simulink library "MicDiagWithdBFSOutput"  (R2022b)
settings: Solver=VariableStepAuto  StartTime=0.0  StopTime=10.0  RelTol=1e-3
values from neighbouring files (symbols this model uses):
  numMicIn = 2    [PhaseDetector_init.m]
undefined symbols (not defined in the file or in its folder): framesize
libraries: RTC x2, FeaturePath x1
settings Model: Creator=pk47312  LastModifiedBy=jk1043656
settings SolverCC: AlgebraicLoopSolver=TrustRegion
settings DebuggingCC: UnconnectedInputMsg=warning  UnconnectedOutputMsg=warning  UnconnectedLineMsg=warning  SFMachineParentedDataDiag=warning
settings ModelReferenceCC: EnableRefExpFcnMdlSchedulingChecks=on
settings RTWCC: DLArmComputeVersion=19.05

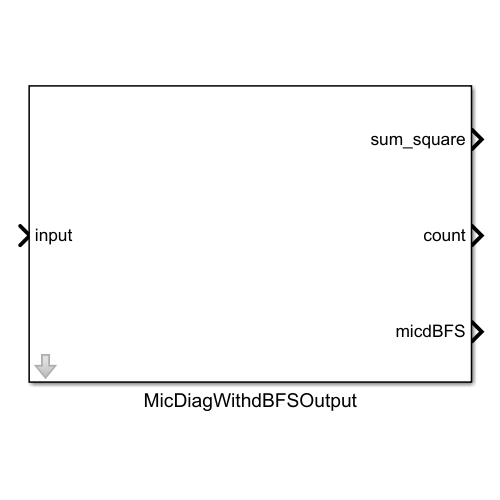
[thumbnail: Simulink's stored preview of the top-level diagram]
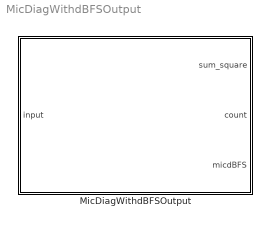
== system MicDiagWithdBFSOutput ==
  MicDiagWithdBFSOutput : Subsystem  mask{numMicIn=numMicIn, framesize=framesize}
      mask prompts: numMicIn "number of Microphone"; framesize "Frame Size"
      mask help: MicDiag accumulates the sum of squares for multiple channels individually

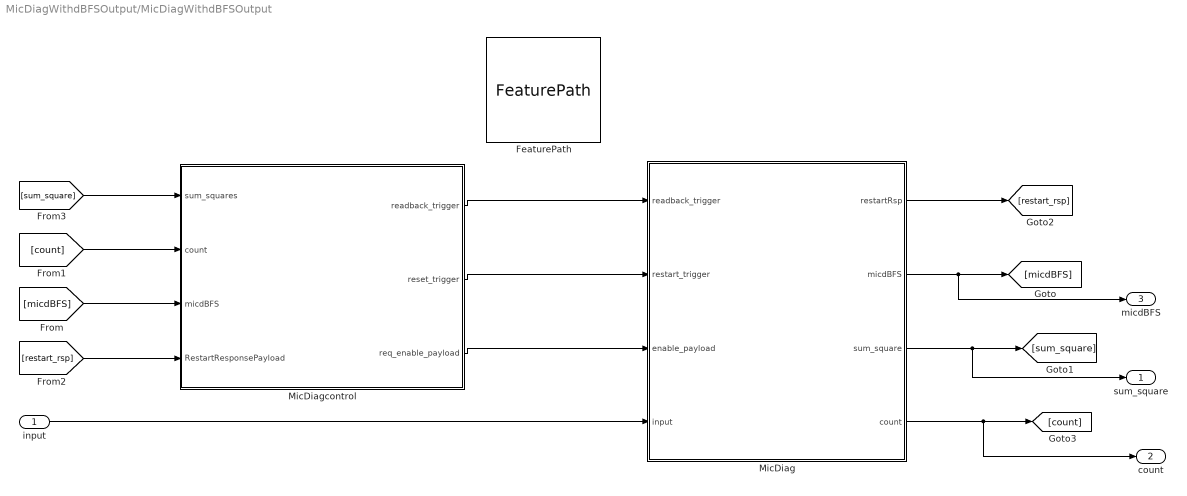
== system MicDiagWithdBFSOutput/MicDiagWithdBFSOutput ==
  input : Inport
  FeaturePath : FeaturePath/FeaturePath  FeatureName=MicDiagWithdBFSOutput  IsGroup=off  GroupNumber=-1  IsModule=off  TriggerInit=[485 19 600 126]
      settings: SourceProductName=Bose Talaria
  MicDiag : Subsystem
  MicDiagcontrol : Subsystem
  sum_square : Outport
  count : Outport  Port=2
  micdBFS : Outport  Port=3
  wires:
  [restart_rsp] -> MicDiagcontrol/4(RestartResponsePayload)
  MicDiagcontrol/3(req_enable_payload) -> MicDiag/3(enable_payload)
  MicDiag/1(restartRsp) -> [restart_rsp]
  [micdBFS] -> MicDiagcontrol/3(micdBFS)
  MicDiagcontrol/1(readback_trigger) -> MicDiag/1(readback_trigger)
  MicDiagcontrol/2(reset_trigger) -> MicDiag/2(restart_trigger)
  input/1 -> MicDiag/4(input)
  MicDiag/2(micdBFS) -> micdBFS/1, [micdBFS]
  MicDiag/3(sum_square) -> sum_square/1, [sum_square]
  MicDiag/4(count) -> count/1, [count]
  [count] -> MicDiagcontrol/2(count)
  [sum_square] -> MicDiagcontrol/1(sum_squares)

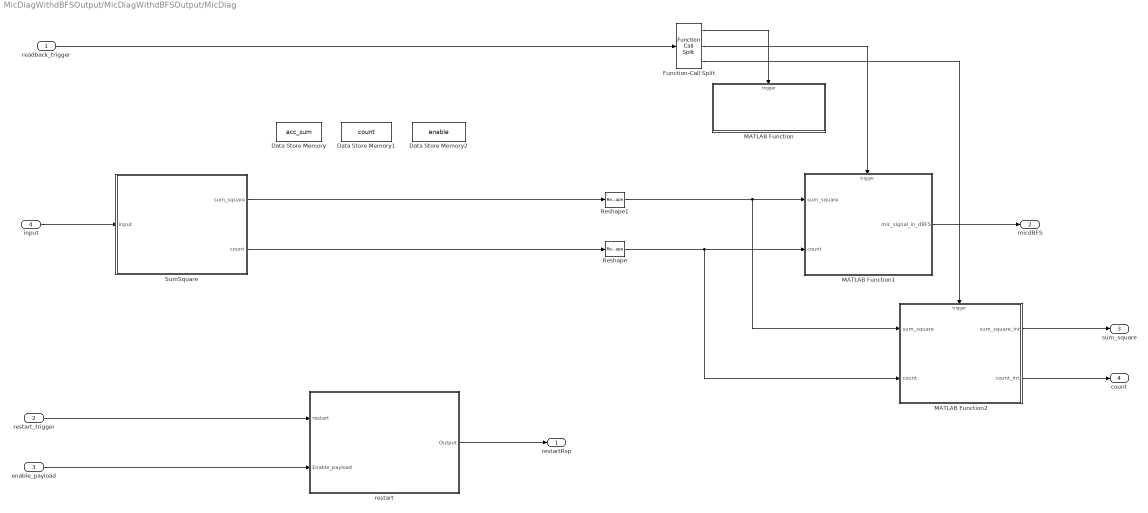
== system MicDiagWithdBFSOutput/MicDiagWithdBFSOutput/MicDiag ==
  readback_trigger : Inport
  restart_trigger : Inport  Port=2
  enable_payload : Inport  Port=3
  input : Inport  Port=4  OutDataTypeStr=single
  Data Store Memory : DataStoreMemory  DataStoreName=acc_sum  InitialValue=zeros(numMicIn,1)  ShowAdditionalParam=off  OutDataTypeStr=single
  Data Store Memory1 : DataStoreMemory  DataStoreName=count  InitialValue=zeros(numMicIn,1)  ShowAdditionalParam=off  OutDataTypeStr=int32
  Data Store Memory2 : DataStoreMemory  DataStoreName=enable  InitialValue=zeros(numMicIn,1)  ShowAdditionalParam=off  OutDataTypeStr=int32
  Function-Call Split : FunctionCallSplit  IconShape=distinctive  NumOutputPorts=3
  MATLAB Function : MATLAB Function  TreatAsAtomicUnit=on
  MATLAB Function1 : MATLAB Function  TreatAsAtomicUnit=on
  MATLAB Function2 : MATLAB Function  TreatAsAtomicUnit=on
  Reshape : Reshape  OutputDimensionality=Row vector (2-D)
  Reshape1 : Reshape  OutputDimensionality=Row vector (2-D)
  SumSquare : Subsystem
  restart : Subsystem
  restartRsp : Outport
  micdBFS : Outport  Port=2  OutDataTypeStr=single
  sum_square : Outport  Port=3  OutDataTypeStr=uint32
  count : Outport  Port=4  OutDataTypeStr=uint32
  wires:
  restart/1(Output) -> restartRsp/1
  Function-Call Split/1 -> MATLAB Function/Trigger
  Function-Call Split/2 -> MATLAB Function1/Trigger
  readback_trigger/1 -> Function-Call Split/1
  input/1 -> SumSquare/1(input)
  restart_trigger/1 -> restart/1(restart)
  enable_payload/1 -> restart/2(Enable_payload)
  SumSquare/1(sum_square) -> Reshape1/1
  SumSquare/2(count) -> Reshape/1
  Reshape1/1 -> MATLAB Function2/1(sum_square), MATLAB Function1/1(sum_square)
  Reshape/1 -> MATLAB Function2/2(count), MATLAB Function1/2(count)
  MATLAB Function1/1(mic_signal_in_dBFS) -> micdBFS/1
  MATLAB Function2/1(sum_square_int) -> sum_square/1
  MATLAB Function2/2(count_int) -> count/1
  Function-Call Split/3 -> MATLAB Function2/Trigger

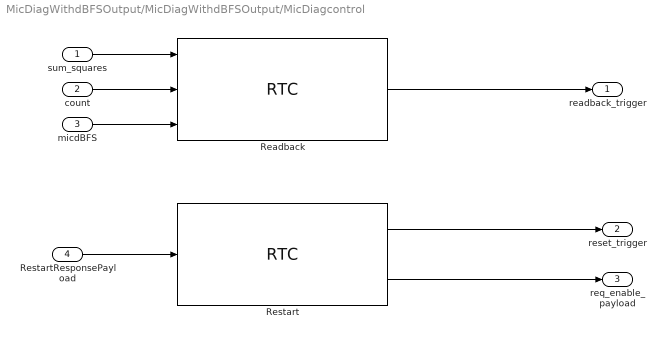
== system MicDiagWithdBFSOutput/MicDiagWithdBFSOutput/MicDiagcontrol ==
  sum_squares : Inport
  count : Inport  Port=2
  micdBFS : Inport  Port=3
  RestartResponsePayload : Inport  Port=4
  Readback : RTC/RTC  REQ_Priority=RTC_Mask.NormalPriority  RequestAtInit=off  EnableRequest=on  REQElemType1=uint32  REQElemWidth1=1  REQElemInitial1=[]  REQElemType2=uint32  REQElemWidth2=1  REQElemInitial2=[]  REQElemType3=uint32  REQElemWidth3=1  REQElemInitial3=[]  REQElemType4=uint32  REQElemWidth4=1  REQElemInitial4=[]  REQElemType5=uint32  REQElemWidth5=1  REQElemInitial5=[]  REQElemType6=uint32  REQElemWidth6=1  REQElemInitial6=[]  REQElemType7=uint32  REQElemWidth7=1  REQElemInitial7=[]  REQElemType8=uint32  REQElemWidth8=1  REQElemInitial8=[]  REQElemType9=uint32  REQElemWidth9=1  REQElemInitial9=[]  REQElemType10=uint32  REQElemWidth10=1  REQElemInitial10=[]  EnableResponse=on  EnableRSP_StatusIn=off  RSPElemName1=sum_squares  RSPElemType1=uint32  RSPElemWidth1=numMicIn  RSPElemName2=count  RSPElemType2=uint32  RSPElemWidth2=numMicIn  RSPElemName3=micdBFS  RSPElemType3=single  RSPElemWidth3=numMicIn  RSPElemType4=uint32  RSPElemWidth4=1  RSPElemType5=uint32  RSPElemWidth5=1  RSPElemType6=uint32  RSPElemWidth6=1  RSPElemType7=uint32  RSPElemWidth7=1  RSPElemType8=uint32  RSPElemWidth8=1  RSPElemType9=uint32  RSPElemWidth9=1  RSPElemType10=uint32  RSPElemWidth10=1  EnableNotification=off  EnableNTF_PrepTrig=off  NTFElemType1=uint32  NTFElemWidth1=1  NTFElemType2=uint32  NTFElemWidth2=1  NTFElemType3=uint32  NTFElemWidth3=1  NTFElemType4=uint32  NTFElemWidth4=1  NTFElemType5=uint32  NTFElemWidth5=1  NTFElemType6=uint32  NTFElemWidth6=1  NTFElemType7=uint32  NTFElemWidth7=1  NTFElemType8=uint32  NTFElemWidth8=1  NTFElemType9=uint32  NTFElemWidth9=1  NTFElemType10=uint32  NTFElemWidth10=1  MaskMessageName=Readback
      settings: SourceProductName=Bose Talaria
  Restart : RTC/RTC  REQ_Priority=RTC_Mask.NormalPriority  RequestAtInit=off  EnableRequest=on  REQElemName1=enable  REQElemType1=int32  REQElemWidth1=numMicIn  REQElemInitial1=[]  REQElemType2=uint32  REQElemWidth2=1  REQElemInitial2=[]  REQElemType3=uint32  REQElemWidth3=1  REQElemInitial3=[]  REQElemType4=uint32  REQElemWidth4=1  REQElemInitial4=[]  REQElemType5=uint32  REQElemWidth5=1  REQElemInitial5=[]  REQElemType6=uint32  REQElemWidth6=1  REQElemInitial6=[]  REQElemType7=uint32  REQElemWidth7=1  REQElemInitial7=[]  REQElemType8=uint32  REQElemWidth8=1  REQElemInitial8=[]  REQElemType9=uint32  REQElemWidth9=1  REQElemInitial9=[]  REQElemType10=uint32  REQElemWidth10=1  REQElemInitial10=[]  EnableResponse=on  EnableRSP_StatusIn=off  RSPElemName1=RestartResponsePayload  RSPElemType1=int32  RSPElemWidth1=1  RSPElemType2=uint32  RSPElemWidth2=1  RSPElemType3=uint32  RSPElemWidth3=1  RSPElemType4=uint32  RSPElemWidth4=1  RSPElemType5=uint32  RSPElemWidth5=1  RSPElemType6=uint32  RSPElemWidth6=1  RSPElemType7=uint32  RSPElemWidth7=1  RSPElemType8=uint32  RSPElemWidth8=1  RSPElemType9=uint32  RSPElemWidth9=1  RSPElemType10=uint32  RSPElemWidth10=1  EnableNotification=off  EnableNTF_PrepTrig=off  NTFElemType1=uint32  NTFElemWidth1=1  NTFElemType2=uint32  NTFElemWidth2=1  NTFElemType3=uint32  NTFElemWidth3=1  NTFElemType4=uint32  NTFElemWidth4=1  NTFElemType5=uint32  NTFElemWidth5=1  NTFElemType6=uint32  NTFElemWidth6=1  NTFElemType7=uint32  NTFElemWidth7=1  NTFElemType8=uint32  NTFElemWidth8=1  NTFElemType9=uint32  NTFElemWidth9=1  NTFElemType10=uint32  NTFElemWidth10=1  MaskMessageName=Restart
      settings: SourceProductName=Bose Talaria
  readback_trigger : Outport
  reset_trigger : Outport  Port=2
  req_enable_payload : Outport  Port=3
  wires:
  RestartResponsePayload/1 -> Restart/1
  micdBFS/1 -> Readback/3
  Restart/1 -> reset_trigger/1
  Readback/1 -> readback_trigger/1
  Restart/2 -> req_enable_payload/1
  sum_squares/1 -> Readback/1
  count/1 -> Readback/2

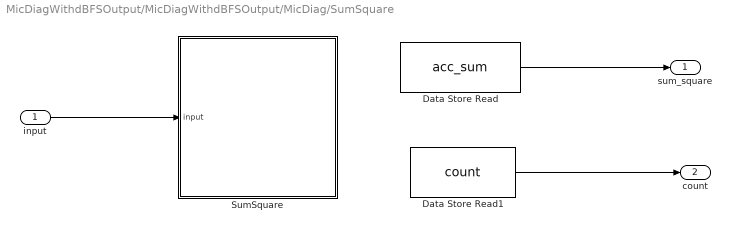
== system MicDiagWithdBFSOutput/MicDiagWithdBFSOutput/MicDiag/SumSquare ==
  input : Inport
  Data Store Read : DataStoreRead  DataStoreName=acc_sum  IndexOptions=Index vector (dialog)  Indices=1  OutputSizes=1
  Data Store Read1 : DataStoreRead  DataStoreName=count  IndexOptions=Index vector (dialog)  Indices=1  OutputSizes=1
  SumSquare : MATLAB Function  TreatAsAtomicUnit=on
  sum_square : Outport
  count : Outport  Port=2
  wires:
  input/1 -> SumSquare/1(input)
  Data Store Read/1 -> sum_square/1
  Data Store Read1/1 -> count/1

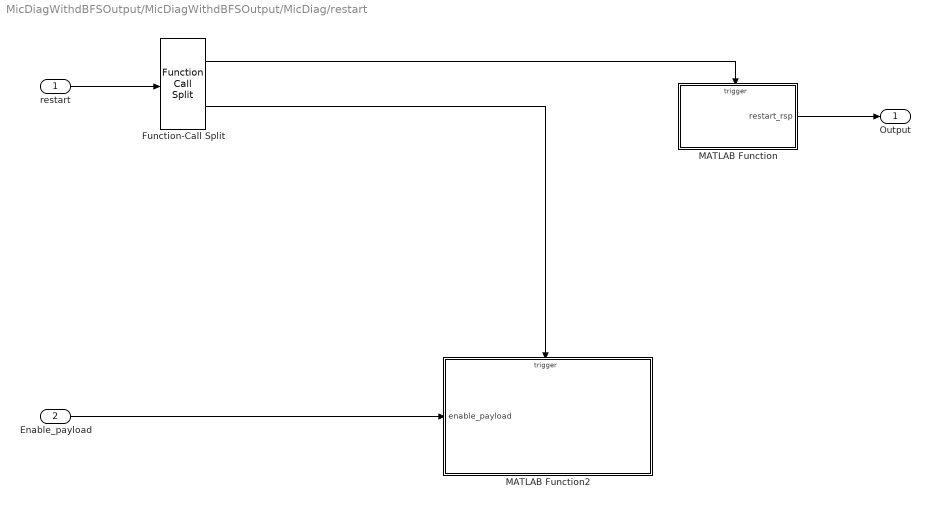
== system MicDiagWithdBFSOutput/MicDiagWithdBFSOutput/MicDiag/restart ==
  restart : Inport
  Enable_payload : Inport  Port=2
  Function-Call Split : FunctionCallSplit  IconShape=distinctive  NumOutputPorts=2  OutputPortLayout=default
  MATLAB Function : MATLAB Function  TreatAsAtomicUnit=on
  MATLAB Function2 : MATLAB Function  TreatAsAtomicUnit=on
  Output : Outport
  wires:
  MATLAB Function/1(restart_rsp) -> Output/1
  Function-Call Split/1 -> MATLAB Function/Trigger
  restart/1 -> Function-Call Split/1
  Function-Call Split/2 -> MATLAB Function2/Trigger
  Enable_payload/1 -> MATLAB Function2/1(enable_payload)

== matlab function MicDiagWithdBFSOutput/MicDiag/MATLAB Function ==
  data: enable data_store_memory
  events: trigger input FUNCTION_CALL_EVENT
function ReadbackDisableAccumulation
    %#codegen
    % datastore memory to control the audio processing logic:
    global enable;
    % find the size of the enable 
    numIn = length(enable);
    % When Readback is requested,accumulation of sum of sqaure shall freeze
    enable = int32(zeros(numIn,1));
end

== matlab function MicDiagWithdBFSOutput/MicDiag/SumSquare/SumSquare ==
  data: input input single size=[framesize numMicIn]; acc_sum data_store_memory; count data_store_memory; enable data_store_memory
function sumsquare(input)
    %#codegen
    % datastore memory to control the audio processing logic:
    global acc_sum;
    global count;
    global enable;
    % number of mic
    numMicIn = size(input,2);
    % frame size
    framesize = size(input,1);
    % Compute sum_of_squares and count
    % if corresponding mic is enabled(which is a RTC message) 
    for MicIn = 1:numMicIn
        if(enable(MicIn) == 1)
            acc_sum(MicIn) = acc_sum(MicIn)+ sum(input(:,MicIn).^2);
            count(MicIn) = count(MicIn)+ framesize;
        end
    end

== matlab function MicDiagWithdBFSOutput/MicDiag/restart/MATLAB Function ==
  data: restart_rsp output int32 size=1
  events: trigger input FUNCTION_CALL_EVENT
function restart_rsp = GenRestartRsp 
% Return the restart reponse as 1
   restart_rsp = int32(1);

== matlab function MicDiagWithdBFSOutput/MicDiag/restart/MATLAB Function2 ==
  data: count data_store_memory; enable data_store_memory; acc_sum data_store_memory; enable_payload input int32 size=numMicIn
  events: trigger input FUNCTION_CALL_EVENT
function restart(enable_payload)
    %#codegen
    % datastore memory to control the audio processing logic:
    global acc_sum;
    global count;
    global enable;
    
    %Fetch the num of the microphone 
    numMicIn  = length(acc_sum);
    
    % freeze the accumulation by clearing enable
    enable = int32(zeros(numMicIn,1));
    % clear accumulator
    acc_sum(1:numMicIn)= single(zeros(numMicIn,1));
    % clear count
    count(1:numMicIn)  = int32(zeros(numMicIn,1));
    
    %unfreeze the accumulation by setting the enable to the paylaod value
    for idx = 1:numMicIn
        if(enable_payload(idx)==1)
            enable(idx) = enable_payload(idx);
        end
    end

== matlab function MicDiagWithdBFSOutput/MicDiag/MATLAB Function1 ==
  data: sum_square input single; mic_signal_in_dBFS output single; count input
  events: trigger input FUNCTION_CALL_EVENT
function mic_signal_in_dBFS = calculate_mic_dbfs(sum_square, count)
Eps = 1e-7;
maxRMSindB = 3.0103; % abs(db20(1/sqrt(2)))
numMicIn = size(sum_square, 2);
micRMS = zeros(1, numMicIn);
mic_signal_in_dBFS = single(zeros(1, numMicIn));
for MicIn = 1:numMicIn
    micRMS(MicIn) = sqrt(sum_square(MicIn)/(single(count(MicIn)) + Eps));
    mic_signal_in_dBFS(MicIn) = db20(micRMS(MicIn) + Eps) + maxRMSindB;
    % dbFS cannot be greater than 0.0
    if (mic_signal_in_dBFS(MicIn) > 0.0)
        mic_signal_in_dBFS(MicIn) = 0.0;
    end
    % 0 dBSPL is usually treated as -126.5 dBFS in ASD
    if (mic_signal_in_dBFS(MicIn) < -126.5)
        mic_signal_in_dBFS(MicIn) = -126.5;
    end
end

== matlab function MicDiagWithdBFSOutput/MicDiag/MATLAB Function2 ==
  data: sum_square input single; sum_square_int output; count input; count_int output
  events: trigger input FUNCTION_CALL_EVENT
function [sum_square_int, count_int] = convert_to_integer(sum_square, count)
sum_square_int = uint32(sum_square);
count_int = uint32(count);
end
